simulink model "dual_pump_actuator_ctrl_OK3"  (R2020a)
settings: Solver=daessc  StartTime=0.0  StopTime=200  MaxStep=tsample
libraries: nesl_utility x12, fl_lib x10, fixed_displacement_pump_lib x2, cstblocks x2, pi_ctrl_lib x1, bichamber_piston_lib x1
settings Model: SimulationMode=accelerator  Creator=dbagn  LastModifiedBy=dabagnara
settings SolverCC: ZeroCrossControl=DisableAll  ZeroCrossAlgorithm=Adaptive
settings DataIOCC: SaveTime=off  ReturnWorkspaceOutputs=off
settings DebuggingCC: IgnoredZcDiagnostic=none
settings SFSimCC: SimParseCustomCode=off

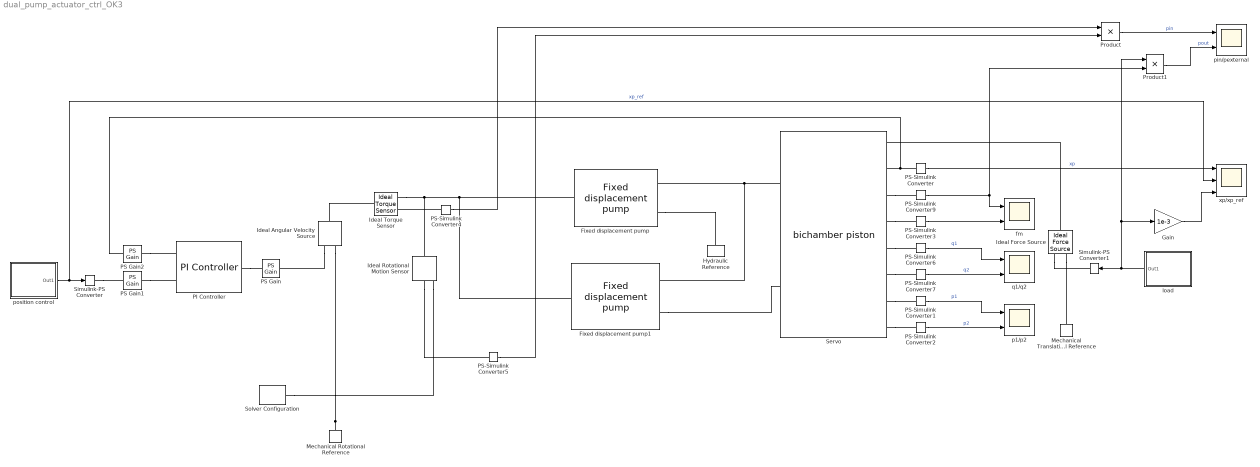
== system dual_pump_actuator_ctrl_OK3 ==
  Fixed displacement pump : fixed_displacement_pump_lib/Fixed displacement pump  max_Dv=100 cm^3/rev  inertia_pump=5e-3 kg*m^2  oil_vol=1 l  bp=0.25 N*m/(rad/s)  lk=1e-6 m  t_specify=off  t_priority=None  t=0 N*m  t_nominal_specify=off  t_nominal_unit=N*m  t_nominal_value=1  q_specify=off  q_priority=None  q=0 m^3/s  q_nominal_specify=off  q_nominal_unit=m^3/s  q_nominal_value=1  qt_specify=off  qt_priority=None  qt=0 m^3/s  qt_nominal_specify=off  qt_nominal_unit=m^3/s  qt_nominal_value=1  qleak_specify=off  qleak_priority=None  qleak=0 m^3/s  qleak_nominal_specify=off  qleak_nominal_unit=m^3/s  qleak_nominal_value=1  Dv_specify=off  Dv_priority=None  Dv=0 cm^3/rev  Dv_nominal_specify=off  Dv_nominal_unit=cm^3/rev  Dv_nominal_value=1  dp_specify=off  dp_priority=None  dp=0 Pa  dp_nominal_specify=off  dp_nominal_unit=Pa  dp_nominal_value=1  we_specify=off  we_priority=None  we=0 rad/s  we_nominal_specify=off  we_nominal_unit=rad/s  we_nominal_value=1
      settings: InternalSimscapePortConfiguration="{\"Bottom\":[],\"Left\":[{\"id\":\"C\",\"label\":\"C\",\"type\":\"foundation.mechanical.rotational.rotational\"}],\"Right\":[{\"id\":\"A\",\"label\":\"A\",\"type\":\"foundation.hydraulic.hydraulic\"},{\"id\":\"B\",\"label\":\"B\",\"type\":\"foundation.hydraulic.hydraulic\"}],\"Top\":[]}"
  Fixed displacement pump1 : fixed_displacement_pump_lib/Fixed displacement pump  max_Dv=100 cm^3/rev  inertia_pump=5e-3 kg*m^2  oil_vol=1 l  bp=0.25 N*m/(rad/s)  lk=1e-6 m  t_specify=off  t_priority=None  t=0 N*m  t_nominal_specify=off  t_nominal_unit=N*m  t_nominal_value=1  q_specify=off  q_priority=None  q=0 m^3/s  q_nominal_specify=off  q_nominal_unit=m^3/s  q_nominal_value=1  qt_specify=off  qt_priority=None  qt=0 m^3/s  qt_nominal_specify=off  qt_nominal_unit=m^3/s  qt_nominal_value=1  qleak_specify=off  qleak_priority=None  qleak=0 m^3/s  qleak_nominal_specify=off  qleak_nominal_unit=m^3/s  qleak_nominal_value=1  Dv_specify=off  Dv_priority=None  Dv=0 cm^3/rev  Dv_nominal_specify=off  Dv_nominal_unit=cm^3/rev  Dv_nominal_value=1  dp_specify=off  dp_priority=None  dp=0 Pa  dp_nominal_specify=off  dp_nominal_unit=Pa  dp_nominal_value=1  we_specify=off  we_priority=None  we=0 rad/s  we_nominal_specify=off  we_nominal_unit=rad/s  we_nominal_value=1
      settings: InternalSimscapePortConfiguration="{\"Bottom\":[],\"Left\":[{\"id\":\"C\",\"label\":\"C\",\"type\":\"foundation.mechanical.rotational.rotational\"}],\"Right\":[{\"id\":\"A\",\"label\":\"A\",\"type\":\"foundation.hydraulic.hydraulic\"},{\"id\":\"B\",\"label\":\"B\",\"type\":\"foundation.hydraulic.hydraulic\"}],\"Top\":[]}"
  Gain : Gain  Gain=1e-3
  Hydraulic Reference : fl_lib/Hydraulic/Hydraulic Elements/Hydraulic Reference
  Ideal Angular Velocity Source : fl_lib/Mechanical/Mechanical Sources/Ideal Angular Velocity Source
  Ideal Force Source : fl_lib/Mechanical/Mechanical Sources/Ideal Force Source
  Ideal Rotational Motion Sensor : fl_lib/Mechanical/Mechanical Sensors/Ideal Rotational Motion Sensor  wrap_angle=simscape.enum.onoff.off  offset=0 rad
  Ideal Torque Sensor : fl_lib/Mechanical/Mechanical Sensors/Ideal Torque Sensor
  Mechanical Rotational Reference : fl_lib/Mechanical/Rotational Elements/Mechanical Rotational Reference
  Mechanical Translational Reference : fl_lib/Mechanical/Translational Elements/Mechanical Translational Reference
  PI Controller : pi_ctrl_lib/PI Controller  kp=20  ki=0 1/s  lim_up=1  lim_bottom=-1  t_ctrl_i_specify=off  t_ctrl_i_priority=None  t_ctrl_i=0  t_ctrl_i_nominal_specify=off  t_ctrl_i_nominal_unit=1  t_ctrl_i_nominal_value=1  t_ctrl_p_specify=off  t_ctrl_p_priority=None  t_ctrl_p=0  t_ctrl_p_nominal_specify=off  t_ctrl_p_nominal_unit=1  t_ctrl_p_nominal_value=1  t_ctrl_out_specify=off  t_ctrl_out_priority=None  t_ctrl_out=0  t_ctrl_out_nominal_specify=off  t_ctrl_out_nominal_unit=1  t_ctrl_out_nominal_value=1  err_specify=off  err_priority=None  err=0  err_nominal_specify=off  err_nominal_unit=1  err_nominal_value=1
      settings: InternalSimscapePortConfiguration="{\"Bottom\":[],\"Left\":[{\"id\":\"meas\",\"label\":\"meas\",\"type\":\"input\"},{\"id\":\"ref\",\"label\":\"ref\",\"type\":\"input\"}],\"Right\":[{\"id\":\"out\",\"label\":\"out\",\"type\":\"output\"}],\"Top\":[]}"
  PS Gain : fl_lib/Physical Signals/Functions/PS Gain  gain=350 rpm
  PS Gain1 : fl_lib/Physical Signals/Functions/PS Gain  gain=1 1/m
  PS Gain2 : fl_lib/Physical Signals/Functions/PS Gain  gain=1 1/m
  PS-Simulink Converter : nesl_utility/PS-Simulink Converter  PhysicalDomain=network_engine_domain  SubClassName=ps_output  LeftPortType=input  RightPortType=output  PseudoPeriodic=off  Frequencies=[]  Unit=m  AffineConversion=on
  PS-Simulink Converter1 : nesl_utility/PS-Simulink Converter  PhysicalDomain=network_engine_domain  SubClassName=ps_output  LeftPortType=input  RightPortType=output  PseudoPeriodic=off  Frequencies=[]  Unit=bar  AffineConversion=on
  PS-Simulink Converter2 : nesl_utility/PS-Simulink Converter  PhysicalDomain=network_engine_domain  SubClassName=ps_output  LeftPortType=input  RightPortType=output  PseudoPeriodic=off  Frequencies=[]  Unit=bar  AffineConversion=on
  PS-Simulink Converter3 : nesl_utility/PS-Simulink Converter  PhysicalDomain=network_engine_domain  SubClassName=ps_output  LeftPortType=input  RightPortType=output  PseudoPeriodic=off  Frequencies=[]  Unit=N  AffineConversion=on
  PS-Simulink Converter4 : nesl_utility/PS-Simulink Converter  PhysicalDomain=network_engine_domain  SubClassName=ps_output  LeftPortType=input  RightPortType=output  PseudoPeriodic=off  Frequencies=[]  Unit=N*m  AffineConversion=on
  PS-Simulink Converter5 : nesl_utility/PS-Simulink Converter  PhysicalDomain=network_engine_domain  SubClassName=ps_output  LeftPortType=input  RightPortType=output  PseudoPeriodic=off  Frequencies=[]  Unit=rad/s  AffineConversion=on
  PS-Simulink Converter6 : nesl_utility/PS-Simulink Converter  PhysicalDomain=network_engine_domain  SubClassName=ps_output  LeftPortType=input  RightPortType=output  PseudoPeriodic=off  Frequencies=[]  Unit=l/min  AffineConversion=on
  PS-Simulink Converter7 : nesl_utility/PS-Simulink Converter  PhysicalDomain=network_engine_domain  SubClassName=ps_output  LeftPortType=input  RightPortType=output  PseudoPeriodic=off  Frequencies=[]  Unit=l/min  AffineConversion=on
  PS-Simulink Converter9 : nesl_utility/PS-Simulink Converter  PhysicalDomain=network_engine_domain  SubClassName=ps_output  LeftPortType=input  RightPortType=output  PseudoPeriodic=off  Frequencies=[]  Unit=m/s  AffineConversion=on
  Product : Product
  Product1 : Product
  Servo : bichamber_piston_lib/bichamber piston  A1=8e-3 m^2  A2=4e-3 m^2  Lp=1 m  mp=35 kg  kp=0 N/m  bp=1e4 N/(m/s)  V0=20 l  q1_specify=off  q1_priority=None  q1=0 m^3/s  q1_nominal_specify=off  q1_nominal_unit=m^3/s  q1_nominal_value=1  q2_specify=off  q2_priority=None  q2=0 m^3/s  q2_nominal_specify=off  q2_nominal_unit=m^3/s  q2_nominal_value=1  p1_specify=off  p1_priority=High  p1=50 bar  p1_nominal_specify=off  p1_nominal_unit=bar  p1_nominal_value=1  p2_specify=off  p2_priority=High  p2=100 bar  p2_nominal_specify=off  p2_nominal_unit=bar  p2_nominal_value=1  fp_specify=off  fp_priority=None  fp=0 N  fp_nominal_specify=off  fp_nominal_unit=N  fp_nominal_value=1  vp_specify=off  vp_priority=High  vp=0 m/s  vp_nominal_specify=off  vp_nominal_unit=m/s  vp_nominal_value=1  xp_specify=off  xp_priority=High  xp=0 m  xp_nominal_specify=off  xp_nominal_unit=m  xp_nominal_value=1
      settings: InternalSimscapePortConfiguration="{\"Bottom\":[],\"Left\":[{\"id\":\"H1\",\"label\":\"H1\",\"type\":\"foundation.hydraulic.hydraulic\"},{\"id\":\"H2\",\"label\":\"H2\",\"type\":\"foundation.hydraulic.hydraulic\"}],\"Right\":[{\"id\":\"P\",\"label\":\"P\",\"type\":\"foundation.mechanical.translational.translational\"},{\"id\":\"xp_out\",\"label\":\"xp\",\"type\":\"output\"},{\"id\":\"vp_out\",\"label\":\"vp\",\"type\":\"output\"},{\"id\":\"mforce\",\"label\":\"fm\",\"type\":\"output\"},{\"id\":\"q1_out\",\"label\":\"q1\",\"type\":\"output\"},{\"id\":\"q2_out\",\"label\":\"q2\",\"type\":\"output\"},{\"id\":\"p1_out\",\"label\":\"p1\",\"type\":\"output\"},{\"id\":\"p2_out\",\"label\":\"p2\",\"type\":\"output\"}],\"Top\":[]}"
  Simulink-PS Converter : nesl_utility/Simulink-PS Converter  PhysicalDomain=network_engine_domain  SubClassName=ps_input  LeftPortType=input  RightPortType=output  PseudoPeriodic=off  Frequencies=[]  NoiseDistribution=none  NoiseParameters=[]  Unit=m  AffineConversion=on  FilteringAndDerivatives=provide  SimscapeFilterOrder=1  InputFilterTimeConstant=0.001  UdotUserProvided=0
  Simulink-PS Converter1 : nesl_utility/Simulink-PS Converter  PhysicalDomain=network_engine_domain  SubClassName=ps_input  LeftPortType=input  RightPortType=output  PseudoPeriodic=off  Frequencies=[]  NoiseDistribution=none  NoiseParameters=[]  Unit=N  AffineConversion=on  FilteringAndDerivatives=provide  SimscapeFilterOrder=1  InputFilterTimeConstant=0.001  UdotUserProvided=0
  Solver Configuration : nesl_utility/Solver Configuration  PhysicalDomain=network_engine_domain  SubClassName=solver  LeftPortType=input  RightPortType=generic  Tones=[]  Harmonics=[]  SimulateNoise=off  Profile=off  UseLocalSampling=off  EnableSwitchedLinearOptims=on  FrequencyDomain=off  UseCCode=off  RelTol=0.001  AbsTol=1e-06  MinStep=1e-09  ToWorkspace=off  RevertToSquareIcSolve=off  NumHomotopyIterations=100  PhasorMode=off  PhasorModeNumHarmonics=1  DoDC=off  ResidualTolerance=1e-09  UseLocalSolver=on  LocalSolverChoice=NE_BACKWARD_EULER_ADVANCER  LocalSolverSampleTime=tsample  DoFixedCost=on  MaxNonlinIter=3  MaxModeIter=2  LinearAlgebra=auto  EquationFormulation=NE_TIME_EF  DelaysMemoryBudget=1024  AutomaticFiltering=on  FilteringTimeConstant=tsample  PartitionStorageMethod=AS_NEEDED  PartitionMemoryBudget=1024  PartitionMethod=ROBUST
  fm : Scope  NumInputPorts=2
  load : Subsystem
  p1/p2 : Scope  NumInputPorts=2
  pin/pexternal : Scope  NumInputPorts=2
  position control : Subsystem
  q1/q2 : Scope  NumInputPorts=2
  xp/xp_ref : Scope  NumInputPorts=3
  wires:
  PS-Simulink Converter1/1 -> p1/p2/1  "p1"
  PS-Simulink Converter2/1 -> p1/p2/2  "p2"
  PS-Simulink Converter3/1 -> fm/2
  PS-Simulink Converter/1 -> xp/xp_ref/1  "xp"
  position control/1(Out1) -> xp/xp_ref/2, Simulink-PS Converter/1  "xp_ref"
  PS-Simulink Converter4/1 -> Product/1
  PS-Simulink Converter5/1 -> Product/2
  load/1(Out1) -> Simulink-PS Converter1/1, Product1/1, Gain/1
  PS-Simulink Converter7/1 -> q1/q2/2  "q2"
  PS-Simulink Converter6/1 -> q1/q2/1  "q1"
  Product/1 -> pin/pexternal/1  "pin"
  Gain/1 -> xp/xp_ref/3
  PS-Simulink Converter9/1 -> fm/1, Product1/2
  Product1/1 -> pin/pexternal/2  "pout"
  connections:
  PS-Simulink Converter/LConn1 -- PS Gain2/LConn1 -- Servo/RConn2
  Servo/RConn7 -- PS-Simulink Converter1/LConn1
  Servo/RConn8 -- PS-Simulink Converter2/LConn1
  Servo/RConn4 -- PS-Simulink Converter3/LConn1
  PI Controller/RConn1 -- PS Gain/LConn1
  Simulink-PS Converter/RConn1 -- PS Gain1/LConn1
  Mechanical Rotational Reference/LConn1 -- Ideal Angular Velocity Source/RConn2 -- Ideal Rotational Motion Sensor/RConn1 -- Solver Configuration/RConn1
  PS Gain1/RConn1 -- PI Controller/LConn2
  PS Gain2/RConn1 -- PI Controller/LConn1
  Ideal Rotational Motion Sensor/RConn2 -- PS-Simulink Converter5/LConn1
  Servo/RConn5 -- PS-Simulink Converter6/LConn1
  Servo/RConn6 -- PS-Simulink Converter7/LConn1
  Fixed displacement pump/RConn2 -- Hydraulic Reference/LConn1
  Fixed displacement pump1/RConn2 -- Servo/LConn2
  Ideal Angular Velocity Source/RConn1 -- PS Gain/RConn1
  Ideal Force Source/LConn1 -- Servo/RConn1
  Ideal Force Source/RConn2 -- Mechanical Translational Reference/LConn1
  Ideal Force Source/RConn1 -- Simulink-PS Converter1/RConn1
  Ideal Rotational Motion Sensor/LConn1 -- Ideal Torque Sensor/RConn1 -- Fixed displacement pump1/LConn1 -- Fixed displacement pump/LConn1
  Servo/RConn3 -- PS-Simulink Converter9/LConn1
  Ideal Angular Velocity Source/LConn1 -- Ideal Torque Sensor/LConn1
  PS-Simulink Converter4/LConn1 -- Ideal Torque Sensor/RConn2
  Servo/LConn1 -- Fixed displacement pump1/RConn1 -- Fixed displacement pump/RConn1

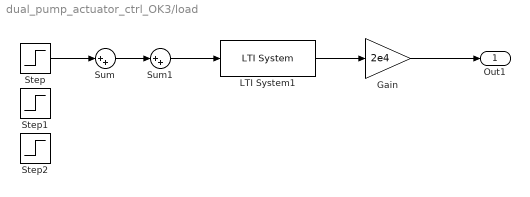
== system dual_pump_actuator_ctrl_OK3/load ==
  Gain : Gain  Gain=2e4
  LTI System1 : cstblocks/LTI System  sys=ref_filter_ss  IC=0
  Step : Step  Time=10  SampleTime=0
  Step1 : Step  Time=60  After=-2  SampleTime=0
  Step2 : Step  Time=125  After=0.25  SampleTime=0
  Sum : Sum  Inputs=|++
  Sum1 : Sum  Inputs=|++
  Out1 : Outport
  wires:
  Step/1 -> Sum/1
  Sum/1 -> Sum1/1
  Gain/1 -> Out1/1
  Sum1/1 -> LTI System1/1
  LTI System1/1 -> Gain/1

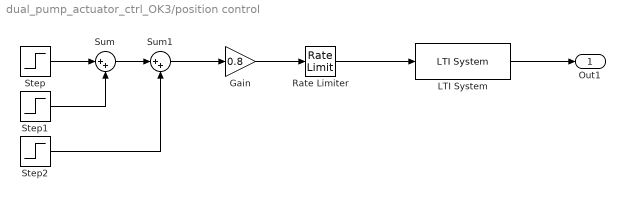
== system dual_pump_actuator_ctrl_OK3/position control ==
  Gain : Gain  Gain=0.8
  LTI System : cstblocks/LTI System  sys=ref_filter_ss  IC=0
  Rate Limiter : RateLimiter  RisingSlewLimit=0.05  FallingSlewLimit=-0.05  SampleTimeMode=inherited
  Step : Step  Time=20  SampleTime=0
  Step1 : Step  Time=60  After=-2  SampleTime=0
  Step2 : Step  Time=125  After=2  SampleTime=0
  Sum : Sum  Inputs=|++
  Sum1 : Sum  Inputs=|++
  Out1 : Outport
  wires:
  Step/1 -> Sum/1
  Sum/1 -> Sum1/1
  Step1/1 -> Sum/2
  Step2/1 -> Sum1/2
  LTI System/1 -> Out1/1
  Rate Limiter/1 -> LTI System/1
  Sum1/1 -> Gain/1
  Gain/1 -> Rate Limiter/1
